simulink model "ECS_FOS"  (Simulink 8.2)
settings: Solver=ode45  StartTime=0.0  StopTime=18000  RelTol=1e-3
InitFcn:
  | load('loss_coeff_mixing_junction.mat')
  | load('SampleOutput.mat')
  | load('HydProp.mat')
  | load('HydraulicLoad.mat')
  | load('initavload.mat')
  | load('SampleFuelBurn.mat')
values from neighbouring files (symbols this model uses):
  FuelBurn = [0 0 0 0 0 0 0 0 0 0 0 0 ... (18249 elements, 1x18249)]    [Benchmark_data1.mat]
  fueltankdata =     [Benchmark_data1.mat]
undefined symbols (not defined in the file or in its folder): AirProp, F1, F2, HUGHES_TREITLER, magnitude, PN_70147, PumpProp
libraries: PowerFlowLib x46, simulink x4
(part 3 of 5)

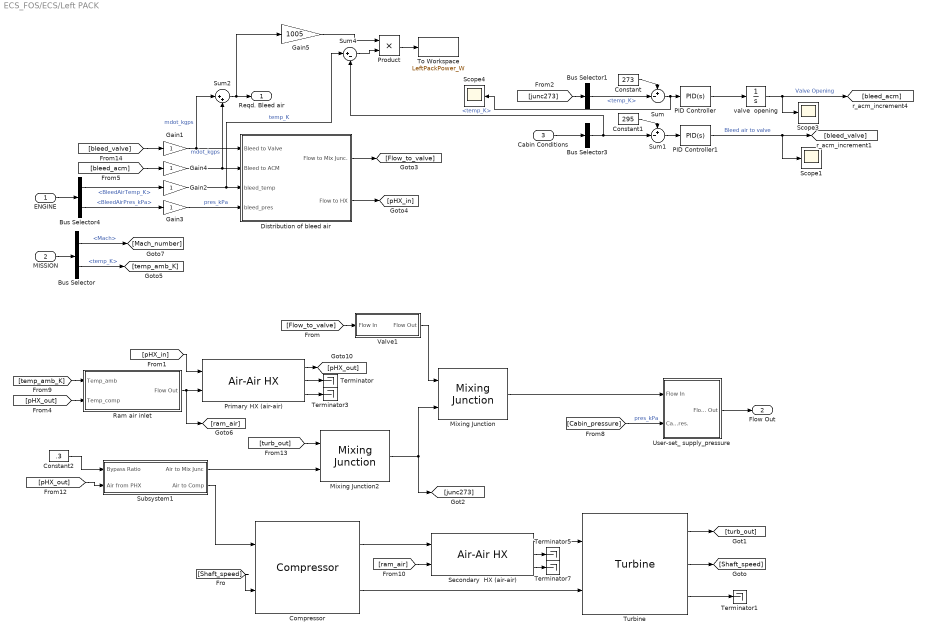
== system ECS_FOS/ECS/Left PACK ==
  ENGINE : Inport
  MISSION : Inport  Port=2
  Cabin Conditions : Inport  Port=3
  Bus Selector : BusSelector  OutputSignals=Flight parameters.Mach,Flight parameters.temp_K
  Bus Selector1 : BusSelector  OutputSignals=temp_K
  Bus Selector3 : BusSelector  OutputSignals=temp_K
  Bus Selector4 : BusSelector  OutputSignals=Bleed.BleedAirTemp_K,Bleed.BleedAirPres_kPa
  Compressor : PowerFlowLib/Energy & Power Systems/Thermal/ECS/Compressor
  Constant : Constant  Value=273
  Constant1 : Constant  Value=295
  Constant2 : Constant  Value=.3
  Distribution of bleed air : Subsystem
      mask Display:
      | port_label('input',1,'{ \bfBleed air to valve [kg/s]}','texmode','on')
      | port_label('input',2,'{ \bfBleed air to ACM [kg/s]}','texmode','on')
      | port_label('input',3,'{ \bfBleed temp. (K)}','texmode','on');
      | port_label('input',4,'{ \bfBleed pressure. (kPa)}','texmode','on')
      | 
      | 
      | 
      | port_label('output',1,'{\bfFlow to Mix Junc. }','texmode','on')
      | port_label('output',2,'{\bfFlow to ACM }','texmode','on')
  Gain{1..4} (4 alike) : Gain
  Gain5 : Gain  Gain=1005
  Mixing Junction : PowerFlowLib/Energy & Power Systems/Thermal/ECS/Mixing Junction  d_in_1=0.1  d_in_2=0.1  d_out=0.2
  Mixing Junction2 : PowerFlowLib/Energy & Power Systems/Thermal/ECS/Mixing Junction  d_in_1=0.1  d_in_2=0.1  d_out=0.2
  PID Controller : simulink/Continuous/PID Controller  Controller=PID  TimeDomain=Continuous-time  SampleTime=1  IntegratorMethod=Forward Euler  FilterMethod=Forward Euler  Form=Parallel  P=.01  I=0  D=0  N=100  InitialConditionSource=internal  InitialConditionForIntegrator=0  InitialConditionForFilter=0  ExternalReset=none  LimitOutput=off  UpperSaturationLimit=inf  LowerSaturationLimit=-inf  LinearizeAsGain=off  AntiWindupMode=none  Kb=1  TrackingMode=off  Kt=1  PParamMin=[]  PParamMax=[]  IParamMin=[]  IParamMax=[]  DParamMin=[]  DParamMax=[]  NParamMin=[]  NParamMax=[]  KbParamMin=[]  KbParamMax=[]  KtParamMin=[]  KtParamMax=[]  POutMin=[]  POutMax=[]  IOutMin=[]  IOutMax=[]  DOutMin=[]  DOutMax=[]  NOutMin=[]  NOutMax=[]  KbOutMin=[]  KbOutMax=[]  KtOutMin=[]  KtOutMax=[]  IntegratorOutMin=[]  IntegratorOutMax=[]  FilterOutMin=[]  FilterOutMax=[]  SumOutMin=[]  SumOutMax=[]  SumI1OutMin=[]  SumI1OutMax=[]  SumI2OutMin=[]  SumI2OutMax=[]  SumI3OutMin=[]  SumI3OutMax=[]  SumDOutMin=[]  SumDOutMax=[]  SaturationOutMin=[]  SaturationOutMax=[]  IntegratorContinuousStateAttributes=''  IntegratorStateMustResolveToSignalObject=off  IntegratorRTWStateStorageClass=Auto  FilterContinuousStateAttributes=''  FilterStateMustResolveToSignalObject=off  FilterRTWStateStorageClass=Auto
  PID Controller1 : simulink/Continuous/PID Controller  Controller=PID  TimeDomain=Continuous-time  SampleTime=1  IntegratorMethod=Forward Euler  FilterMethod=Forward Euler  Form=Parallel  P=.2  I=.01  D=0  N=100  InitialConditionSource=internal  InitialConditionForIntegrator=0  InitialConditionForFilter=0  ExternalReset=none  LimitOutput=on  UpperSaturationLimit=inf  LowerSaturationLimit=.05  LinearizeAsGain=off  AntiWindupMode=none  Kb=1  TrackingMode=off  Kt=1  PParamMin=[]  PParamMax=[]  IParamMin=[]  IParamMax=[]  DParamMin=[]  DParamMax=[]  NParamMin=[]  NParamMax=[]  KbParamMin=[]  KbParamMax=[]  KtParamMin=[]  KtParamMax=[]  POutMin=[]  POutMax=[]  IOutMin=[]  IOutMax=[]  DOutMin=[]  DOutMax=[]  NOutMin=[]  NOutMax=[]  KbOutMin=[]  KbOutMax=[]  KtOutMin=[]  KtOutMax=[]  IntegratorOutMin=[]  IntegratorOutMax=[]  FilterOutMin=[]  FilterOutMax=[]  SumOutMin=[]  SumOutMax=[]  SumI1OutMin=[]  SumI1OutMax=[]  SumI2OutMin=[]  SumI2OutMax=[]  SumI3OutMin=[]  SumI3OutMax=[]  SumDOutMin=[]  SumDOutMax=[]  SaturationOutMin=[]  SaturationOutMax=[]  IntegratorContinuousStateAttributes=''  IntegratorStateMustResolveToSignalObject=off  IntegratorRTWStateStorageClass=Auto  FilterContinuousStateAttributes=''  FilterStateMustResolveToSignalObject=off  FilterRTWStateStorageClass=Auto
  Primary HX (air-air) : PowerFlowLib/Energy & Power Systems/Thermal/ECS/Air-Air HX  L_hx=0.2  W_hx=0.2  H_hx=0.2  t_p=0.0008  K_p=167  cp_hx=883  m_cm=16  l_fin=.005  t_fin=0.0002  s_fin=0.0015  h_fin=0.0095  K_n=167  eta_f=0.8  T_cm_0=50
  Product : Product
  Ram air inlet : Subsystem  mask{ram_air=.5, T_35=273}
      mask prompts: ram_air "Ram air mass flow rate"; T_35 "Temperature control for 35F valve"
      mask Display:
      | port_label('input',1,'{ \bf Ambient Temp.}','texmode','on')
      | port_label('input',2,'{ \bf Comp. Face Temp.}','texmode','on');
      | 
      | port_label('output',1,'{\bf Flow Out}','texmode','on')
  Scope1 : Scope
      settings: YMin=0  YMax=6.5  SaveName=ScopeData33  SampleInput=on  SampleTime=1
  Scope3 : Scope
      settings: YMin=0.735  YMax=0.8  SaveName=ScopeData35  SampleInput=on  SampleTime=1
  Scope4 : Scope
      settings: TimeRange=1500  YMin=2.8421709427e-013  YMax=2.8421709434e-013  SaveName=ScopeData37  SampleInput=on  SampleTime=1
  Secondary  HX (air-air) : PowerFlowLib/Energy & Power Systems/Thermal/ECS/Air-Air HX  L_hx=0.2  W_hx=0.2  H_hx=0.2  t_p=0.0008  K_p=167  cp_hx=883  m_cm=16  l_fin=.005  t_fin=0.0002  s_fin=0.0015  h_fin=0.0095  K_n=167  eta_f=0.8  T_cm_0=25
  Subsystem1 : Subsystem
  Sum : Sum  Inputs=+-|
  Sum1 : Sum  Inputs=+-|
  Sum2 : Sum  Inputs=|++
  Sum4 : Sum  Inputs=|+-
  Terminator{,1,3,5,7} (5 alike) : Terminator
  To Workspace : ToWorkspace  VariableName=LeftPackPower_W  SampleTime=10  SaveFormat=Structure With Time
  Turbine : PowerFlowLib/Energy & Power Systems/Thermal/ECS/Turbine  press_Turbine_exit=80  inertia=5e-5  n_t=0.7
  User-set_ supply_pressure : Subsystem
  Valve1 : Subsystem
  valve  opening : Integrator  InitialCondition=.2  LimitOutput=on  UpperSaturationLimit=.9  LowerSaturationLimit=.2
  Reqd. Bleed air : Outport
  Flow Out : Outport  Port=2
  wires:
  Product/1 -> To Workspace/1
  Sum4/1 -> Product/2
  Gain5/1 -> Product/1
  Constant2/1 -> Subsystem1/1(Bypass Ratio)
  [bleed_acm] -> Gain4/1
  Cabin Conditions/1 -> Bus Selector3/1
  Sum2/1 -> Reqd. Bleed air/1, Gain5/1
  Gain4/1 -> Sum2/2, Distribution of bleed air/2(Bleed to ACM)  "mdot_kgps"
  Constant/1 -> Sum/1
  valve  opening/1 -> [bleed_acm], Scope3/1  "Valve Opening"
  PID Controller/1 -> valve  opening/1
  Sum/1 -> Scope4/1, PID Controller/1
  Bus Selector1/1 -> Sum/2  "<temp_K>"
  [junc273] -> Bus Selector1/1
  Subsystem1/2(Air to Comp) -> Compressor/1
  Subsystem1/1(Air to Mix Junc) -> Mixing Junction2/2
  [turb_out] -> Mixing Junction2/1
  Mixing Junction2/1 -> Mixing Junction/2, [junc273]
  [pHX_out] -> Subsystem1/2(Air from PHX)
  Secondary  HX (air-air)/1 -> Turbine/1
  Secondary  HX (air-air)/3 -> Terminator7/1
  Secondary  HX (air-air)/2 -> Terminator5/1
  Primary HX (air-air)/1 -> [pHX_out]
  Primary HX (air-air)/2 -> Terminator/1
  Primary HX (air-air)/3 -> Terminator3/1
  [bleed_valve] -> Gain1/1
  Gain3/1 -> Distribution of bleed air/4(bleed_pres)  "pres_kPa"
  Gain2/1 -> Distribution of bleed air/3(bleed_temp), Sum4/1  "temp_K"
  Gain1/1 -> Sum2/1, Distribution of bleed air/1(Bleed to Valve)  "mdot_kgps"
  Bus Selector/1 -> [Mach_number]  "<Mach>"
  Bus Selector/2 -> [temp_amb_K]  "<temp_K>"
  Bus Selector4/2 -> Gain3/1  "<BleedAirPres_kPa>"
  Bus Selector4/1 -> Gain2/1  "<BleedAirTemp_K>"
  Distribution of bleed air/1(Flow to Mix Junc.) -> [Flow_to_valve]
  Distribution of bleed air/2(Flow to HX) -> [pHX_in]
  ENGINE/1 -> Bus Selector4/1
  MISSION/1 -> Bus Selector/1
  [pHX_out] -> Ram air inlet/2(Temp_comp)
  [temp_amb_K] -> Ram air inlet/1(Temp_amb)
  [Cabin_pressure] -> User-set_ supply_pressure/2(Cabin Pres.)  "pres_kPa"
  User-set_ supply_pressure/1(Flow Out) -> Flow Out/1
  Turbine/1 -> [turb_out]
  Turbine/3 -> Terminator1/1
  Turbine/2 -> [Shaft_speed]
  Mixing Junction/1 -> User-set_ supply_pressure/1(Flow In)
  [ram_air] -> Secondary  HX (air-air)/2
  Compressor/1 -> Secondary  HX (air-air)/1
  Ram air inlet/1(Flow Out) -> [ram_air], Primary HX (air-air)/2
  Compressor/2 -> Turbine/2
  [Shaft_speed] -> Compressor/2
  [Flow_to_valve] -> Valve1/1(Flow In)
  Valve1/1(Flow Out) -> Mixing Junction/1
  [pHX_in] -> Primary HX (air-air)/1
  Bus Selector3/1 -> Sum1/2, Sum4/2  "<temp_K>"
  Sum1/1 -> PID Controller1/1
  PID Controller1/1 -> Scope1/1, [bleed_valve]  "Bleed air to valve"
  Constant1/1 -> Sum1/1

== system ECS_FOS/ECS/Oil Tanks/Pumps Left Wing ==
  Oil Sys Pres : Inport
  Flow In : Inport  Port=2
  Bus Selector1 : BusSelector  OutputSignals=Oil
  Bus Selector2 : BusSelector  OutputSignals=real_pwr_W,react_pwr_VAr
  Bus Selector5 : BusSelector  OutputSignals=mdot_kgps,pres_kPa
  ElectricalSink1 : PowerFlowLib/Support Functions//Tools/ElectricalSink  Tag=Flow  Description=TwoPhase  load_loc=LeftWing  ACDC_load=AC  units=Watts  unq_id=9405
  Fuel Switch1 : Constant  Value=100
  Fuel Switch2 : Constant  Value=1400
  Fuel Switch3 : Constant  Value=[10 10 10 10 10 10]
  Oil Pump : PowerFlowLib/Energy & Power Systems/Thermal/Oil/Oil Pump  maptype=Pressure (kPa) vs. Vol. Flow Rate (m³/hr)  map=B737_mech_fuel1  map_load=off  SG=0.82  pump_eff=.75  heat_out=off  AC_pwr=on  pf=1  mech_pwr=off
  Oil Tank : Subsystem  AncestorBlock=PowerFlowLib/Energy & Power Systems/Thermal/Fuel/Fuel Tank  mask(Fuel Tank){fileslct=off, filename=fueltank_area.m, filedir=C:\Users\mwillms4\Documents\My Box Files\Graduate\Research\PowerFlow Development\PowerFlow Fall 2013\SupportFunctions\fueltank_area.m, tank_loc=Left Wing Tank, areaprompt2=off, max_vol=3.2, m_init=2500, fld_Tint=0, ull_Tint=30, Pover=100, HTC_fg=14.2, wallHXF=off, wetHTC=14.2, dryHTC=14.2, Qinternal=0}
      mask prompts: fileslct "Browse for area .m file?"; filename "Fuel Tank Area .m File"; filedir "Area .m File Directory"; tank_loc "Select Tank"; areaprompt2 "Edit Fuel Tank Area Manually?"; max_vol "Maximum Tank Volume [m³]"; m_init "Initial Fluid Mass [kg]"; fld_Tint "Initial Fluid Temperature [°C]"; ull_Tint "Initial Ullage Temperature [°C]"; Pover "Tank Pressurization [kPa]"; HTC_fg "Fuel to Ullage HTC [W/m² K]"; wallHXF "Enable Wall Heat Transfer"; wetHTC "Wall to Fluid HTC [W/m² K]"; dryHTC "Wall to Ullage HTC [W/m² K]"; Qinternal "Internal Heat Load [W]"
      mask help:
      | Input 1: Input Flow Bus
      | Input 2: Flow Rate Out [kg/s]
      | Input 3: Ambient Pressure [kPa]
      | Input 4: Heat Load [W]
      | Input 5: Initial Wall Temps. Vector [K]
      |
      | Output 1: Output Flow Bus
      | Output 2: Tank mass [kg]
      | Output 3: Ullage Temp. [K]
      mask init: same as ECS_FOS/ECS/Fuel Tanks/Pumps/Center Fuel Tank
      mask Callback fileslct:
      | h      = get_param(gcb,'handle');   % Get block handle
      | blk    = gcb;
      | hblock = get(h);     % Parse out handles structure
      | 
      | if strcmp(hblock.fileslct,'on') == 1;
      |     set_param(gcb,'areaprompt2','off');     % turn off manual switch
      |     RR_SetPerfSlct(2,0);                    % call uiopen script
      | end
      | 
      | clear h blk hblock
      mask TypeOptions tank_loc: Left Wing Tank | Center Tank | Right Wing Tank
      mask Callback areaprompt2:
      | h      = get_param(gcb,'handle');   % Get block handle
      | blk    = gcb;
      | hblock = get(h);     % Parse out handles structure
      | 
      | if strcmp(hblock.areaprompt2,'on') == 1;
      |     set_param(gcb,'fileslct','off');
      |     open_system([blk, '/Wall Heat Transfer/volume_%']);
      | end
      mask Callback wallHXF:
      | h      = get_param(gcb,'handle');   % Get block handle
      | blk    = gcb;
      | hblock = get(h);     % Parse out handles structure
      | 
      | if strcmp(hblock.wallHXF,'on') == 1;
      |     set_param([blk,'/enable_wall_HXF'],'Value','1');
      | else
      |     set_param([blk,'/enable_wall_HXF'],'Value','0');
      | end
      | 
      | clear h blk hblock
      mask Display:
      | image(imread('fueltank.jpg'))
      | 
      | port_label('input',1,'{\bf Flow In}','TexMode','on')
      | port_label('input',2,'{\bf Flow Rate Out}','TexMode','on')
      | port_label('input',3,'{\bf P_a_m_b [kPa]}','TexMode','on')
      | port_label('input',4,'{\bf Heat Load [kW]}','TexMode','on')
      | port_label('input',5,'{\bf Wall Temp. [K]}','TexMode','on')
      | 
      | port_label('output',1,'{\bf Flow Out }','TexMode','on')
      | port_label('output',2,'{\bf Fluid Mass [kg]}','TexMode','on')
      | port_label('output',3,'{\bf Ullage Temp. [K]}','TexMode','on')
  Terminator : Terminator
  Terminator1 : Terminator
  Oil To HX : Outport
  wires:
  Oil Pump/2 -> Bus Selector2/1
  Bus Selector2/2 -> ElectricalSink1/2  "<react_pwr_VAr>"
  Bus Selector2/1 -> ElectricalSink1/1  "<real_pwr_W>"
  Oil Tank/1(Flow_Out) -> Oil Pump/1
  Oil Tank/2(fluid_mass) -> Terminator/1
  Oil Tank/3(ullage_T) -> Terminator1/1
  Fuel Switch3/1 -> Oil Tank/5(Wall_temps)
  Oil Pump/3 -> Oil Tank/4(Heat load)
  Oil Pump/1 -> Bus Selector5/1, Oil To HX/1
  Fuel Switch1/1 -> Oil Tank/3(Pamb)
  Oil Sys Pres/1 -> Oil Pump/3
  Flow In/1 -> Bus Selector1/1
  Fuel Switch2/1 -> Oil Pump/2
  Bus Selector5/1 -> Oil Tank/2(Flow Out)  "<mdot_kgps>"
  Bus Selector1/1 -> Oil Tank/1(Flow)  "<Oil>"

== system ECS_FOS/ECS/Oil Tanks/Pumps Right Wing ==
  Oil Sys Pres : Inport
  Flow In : Inport  Port=2
  Bus Selector1 : BusSelector  OutputSignals=Oil
  Bus Selector2 : BusSelector  OutputSignals=real_pwr_W,react_pwr_VAr
  Bus Selector5 : BusSelector  OutputSignals=mdot_kgps,pres_kPa
  ElectricalSink1 : PowerFlowLib/Support Functions//Tools/ElectricalSink  Tag=Flow  Description=TwoPhase  load_loc=RightWing  ACDC_load=AC  units=Watts  unq_id=2169
  Fuel Switch2 : Constant  Value=1400
  Fuel Tank : Subsystem  AncestorBlock=PowerFlowLib/Energy & Power Systems/Thermal/Fuel/Fuel Tank  mask(Fuel Tank){fileslct=off, filename=fueltank_area.m, filedir=C:\Users\mwillms4\Documents\My Box Files\Graduate\Research\PowerFlow Development\PowerFlow Fall 2013\SupportFunctions\fueltank_area.m, tank_loc=Left Wing Tank, areaprompt2=off, max_vol=3.2, m_init=2500, fld_Tint=0, ull_Tint=30, Pover=100, HTC_fg=14.2, wallHXF=off, wetHTC=14.2, dryHTC=14.2, Qinternal=0}
      mask prompts: fileslct "Browse for area .m file?"; filename "Fuel Tank Area .m File"; filedir "Area .m File Directory"; tank_loc "Select Tank"; areaprompt2 "Edit Fuel Tank Area Manually?"; max_vol "Maximum Tank Volume [m³]"; m_init "Initial Fluid Mass [kg]"; fld_Tint "Initial Fluid Temperature [°C]"; ull_Tint "Initial Ullage Temperature [°C]"; Pover "Tank Pressurization [kPa]"; HTC_fg "Fuel to Ullage HTC [W/m² K]"; wallHXF "Enable Wall Heat Transfer"; wetHTC "Wall to Fluid HTC [W/m² K]"; dryHTC "Wall to Ullage HTC [W/m² K]"; Qinternal "Internal Heat Load [W]"
      mask help:
      | Input 1: Input Flow Bus
      | Input 2: Flow Rate Out [kg/s]
      | Input 3: Ambient Pressure [kPa]
      | Input 4: Heat Load [W]
      | Input 5: Initial Wall Temps. Vector [K]
      |
      | Output 1: Output Flow Bus
      | Output 2: Tank mass [kg]
      | Output 3: Ullage Temp. [K]
      mask init: same as ECS_FOS/ECS/Fuel Tanks/Pumps/Center Fuel Tank
      mask Callback fileslct:
      | h      = get_param(gcb,'handle');   % Get block handle
      | blk    = gcb;
      | hblock = get(h);     % Parse out handles structure
      | 
      | if strcmp(hblock.fileslct,'on') == 1;
      |     set_param(gcb,'areaprompt2','off');     % turn off manual switch
      |     RR_SetPerfSlct(2,0);                    % call uiopen script
      | end
      | 
      | clear h blk hblock
      mask TypeOptions tank_loc: Left Wing Tank | Center Tank | Right Wing Tank
      mask Callback areaprompt2:
      | h      = get_param(gcb,'handle');   % Get block handle
      | blk    = gcb;
      | hblock = get(h);     % Parse out handles structure
      | 
      | if strcmp(hblock.areaprompt2,'on') == 1;
      |     set_param(gcb,'fileslct','off');
      |     open_system([blk, '/Wall Heat Transfer/volume_%']);
      | end
      mask Callback wallHXF:
      | h      = get_param(gcb,'handle');   % Get block handle
      | blk    = gcb;
      | hblock = get(h);     % Parse out handles structure
      | 
      | if strcmp(hblock.wallHXF,'on') == 1;
      |     set_param([blk,'/enable_wall_HXF'],'Value','1');
      | else
      |     set_param([blk,'/enable_wall_HXF'],'Value','0');
      | end
      | 
      | clear h blk hblock
      mask Display:
      | image(imread('fueltank.jpg'))
      | 
      | port_label('input',1,'{\bf Flow In}','TexMode','on')
      | port_label('input',2,'{\bf Flow Rate Out}','TexMode','on')
      | port_label('input',3,'{\bf P_a_m_b [kPa]}','TexMode','on')
      | port_label('input',4,'{\bf Heat Load [kW]}','TexMode','on')
      | port_label('input',5,'{\bf Wall Temp. [K]}','TexMode','on')
      | 
      | port_label('output',1,'{\bf Flow Out }','TexMode','on')
      | port_label('output',2,'{\bf Fluid Mass [kg]}','TexMode','on')
      | port_label('output',3,'{\bf Ullage Temp. [K]}','TexMode','on')
  Ground : Ground
  Ground1 : Ground
  Oil Pump : PowerFlowLib/Energy & Power Systems/Thermal/Oil/Oil Pump  maptype=Pressure (kPa) vs. Vol. Flow Rate (m³/hr)  map=B737_mech_fuel1  map_load=off  SG=0.82  pump_eff=.75  heat_out=off  AC_pwr=on  pf=1  mech_pwr=off
  Terminator : Terminator
  Terminator1 : Terminator
  Oil To HX : Outport
  wires:
  Bus Selector1/1 -> Fuel Tank/1(Flow)  "<Oil>"
  Oil Pump/2 -> Bus Selector2/1
  Bus Selector2/2 -> ElectricalSink1/2  "<react_pwr_VAr>"
  Bus Selector2/1 -> ElectricalSink1/1  "<real_pwr_W>"
  Bus Selector5/1 -> Fuel Tank/2(Flow Out)  "<mdot_kgps>"
  Fuel Switch2/1 -> Oil Pump/2
  Flow In/1 -> Bus Selector1/1
  Oil Sys Pres/1 -> Oil Pump/3
  Ground1/1 -> Fuel Tank/3(Pamb)
  Oil Pump/1 -> Oil To HX/1, Bus Selector5/1
  Oil Pump/3 -> Fuel Tank/4(Heat load)
  Ground/1 -> Fuel Tank/5(Wall_temps)
  Fuel Tank/3(ullage_T) -> Terminator1/1
  Fuel Tank/2(fluid_mass) -> Terminator/1
  Fuel Tank/1(Flow_Out) -> Oil Pump/1

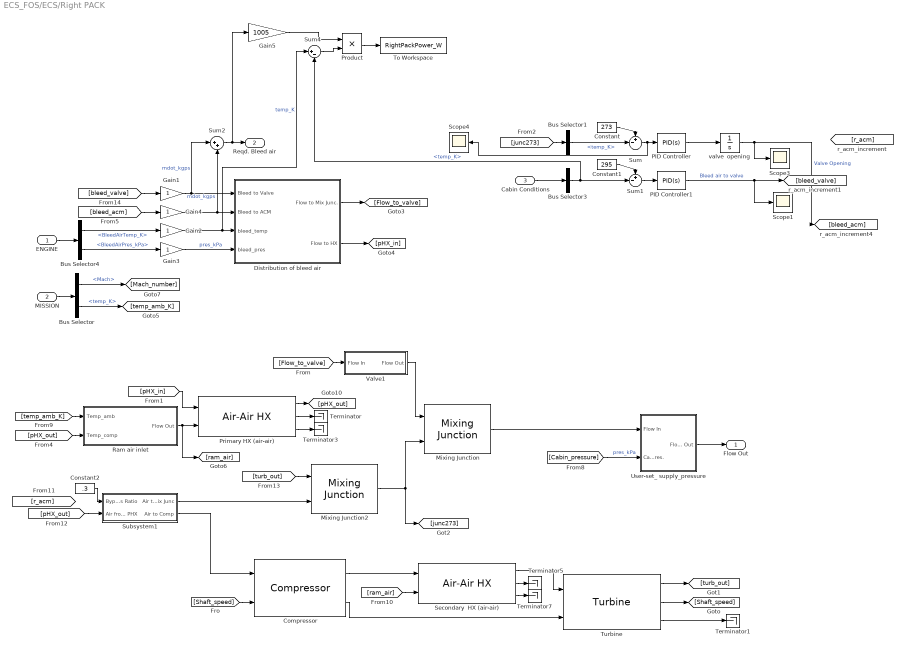
== system ECS_FOS/ECS/Right PACK ==
  ENGINE : Inport
  MISSION : Inport  Port=2
  Cabin Conditions : Inport  Port=3
  Bus Selector : BusSelector  OutputSignals=Flight parameters.Mach,Flight parameters.temp_K
  Bus Selector1 : BusSelector  OutputSignals=temp_K
  Bus Selector3 : BusSelector  OutputSignals=temp_K
  Bus Selector4 : BusSelector  OutputSignals=Bleed.BleedAirTemp_K,Bleed.BleedAirPres_kPa
  Compressor : PowerFlowLib/Energy & Power Systems/Thermal/ECS/Compressor
  Constant : Constant  Value=273
  Constant1 : Constant  Value=295
  Constant2 : Constant  Value=.3
  Distribution of bleed air : Subsystem
      mask Display:
      | port_label('input',1,'{ \bfBleed air to valve [kg/s]}','texmode','on')
      | port_label('input',2,'{ \bfBleed air to ACM [kg/s]}','texmode','on')
      | port_label('input',3,'{ \bfBleed temp. (K)}','texmode','on');
      | port_label('input',4,'{ \bfBleed pressure. (kPa)}','texmode','on')
      | 
      | 
      | 
      | port_label('output',1,'{\bfFlow to Mix Junc. }','texmode','on')
      | port_label('output',2,'{\bfFlow to ACM }','texmode','on')
  Gain{1..4} (4 alike) : Gain
  Gain5 : Gain  Gain=1005
  Mixing Junction : PowerFlowLib/Energy & Power Systems/Thermal/ECS/Mixing Junction  d_in_1=0.1  d_in_2=0.1  d_out=0.2
  Mixing Junction2 : PowerFlowLib/Energy & Power Systems/Thermal/ECS/Mixing Junction  d_in_1=0.1  d_in_2=0.1  d_out=0.2
  PID Controller : simulink/Continuous/PID Controller  Controller=PID  TimeDomain=Continuous-time  SampleTime=1  IntegratorMethod=Forward Euler  FilterMethod=Forward Euler  Form=Parallel  P=.01  I=0  D=0  N=100  InitialConditionSource=internal  InitialConditionForIntegrator=0  InitialConditionForFilter=0  ExternalReset=none  LimitOutput=off  UpperSaturationLimit=inf  LowerSaturationLimit=-inf  LinearizeAsGain=off  AntiWindupMode=none  Kb=1  TrackingMode=off  Kt=1  PParamMin=[]  PParamMax=[]  IParamMin=[]  IParamMax=[]  DParamMin=[]  DParamMax=[]  NParamMin=[]  NParamMax=[]  KbParamMin=[]  KbParamMax=[]  KtParamMin=[]  KtParamMax=[]  POutMin=[]  POutMax=[]  IOutMin=[]  IOutMax=[]  DOutMin=[]  DOutMax=[]  NOutMin=[]  NOutMax=[]  KbOutMin=[]  KbOutMax=[]  KtOutMin=[]  KtOutMax=[]  IntegratorOutMin=[]  IntegratorOutMax=[]  FilterOutMin=[]  FilterOutMax=[]  SumOutMin=[]  SumOutMax=[]  SumI1OutMin=[]  SumI1OutMax=[]  SumI2OutMin=[]  SumI2OutMax=[]  SumI3OutMin=[]  SumI3OutMax=[]  SumDOutMin=[]  SumDOutMax=[]  SaturationOutMin=[]  SaturationOutMax=[]  IntegratorContinuousStateAttributes=''  IntegratorStateMustResolveToSignalObject=off  IntegratorRTWStateStorageClass=Auto  FilterContinuousStateAttributes=''  FilterStateMustResolveToSignalObject=off  FilterRTWStateStorageClass=Auto
  PID Controller1 : simulink/Continuous/PID Controller  Controller=PID  TimeDomain=Continuous-time  SampleTime=1  IntegratorMethod=Forward Euler  FilterMethod=Forward Euler  Form=Parallel  P=.2  I=.01  D=0  N=0  InitialConditionSource=internal  InitialConditionForIntegrator=0  InitialConditionForFilter=0  ExternalReset=none  LimitOutput=on  UpperSaturationLimit=10  LowerSaturationLimit=.05  LinearizeAsGain=off  AntiWindupMode=none  Kb=1  TrackingMode=off  Kt=1  PParamMin=[]  PParamMax=[]  IParamMin=[]  IParamMax=[]  DParamMin=[]  DParamMax=[]  NParamMin=[]  NParamMax=[]  KbParamMin=[]  KbParamMax=[]  KtParamMin=[]  KtParamMax=[]  POutMin=[]  POutMax=[]  IOutMin=[]  IOutMax=[]  DOutMin=[]  DOutMax=[]  NOutMin=[]  NOutMax=[]  KbOutMin=[]  KbOutMax=[]  KtOutMin=[]  KtOutMax=[]  IntegratorOutMin=[]  IntegratorOutMax=[]  FilterOutMin=[]  FilterOutMax=[]  SumOutMin=[]  SumOutMax=[]  SumI1OutMin=[]  SumI1OutMax=[]  SumI2OutMin=[]  SumI2OutMax=[]  SumI3OutMin=[]  SumI3OutMax=[]  SumDOutMin=[]  SumDOutMax=[]  SaturationOutMin=[]  SaturationOutMax=[]  IntegratorContinuousStateAttributes=''  IntegratorStateMustResolveToSignalObject=off  IntegratorRTWStateStorageClass=Auto  FilterContinuousStateAttributes=''  FilterStateMustResolveToSignalObject=off  FilterRTWStateStorageClass=Auto
  Primary HX (air-air) : PowerFlowLib/Energy & Power Systems/Thermal/ECS/Air-Air HX  L_hx=0.2  W_hx=0.2  H_hx=0.2  t_p=0.0008  K_p=167  cp_hx=883  m_cm=16  l_fin=.005  t_fin=0.0002  s_fin=0.0015  h_fin=0.0095  K_n=167  eta_f=0.8  T_cm_0=50
  Product : Product
  Ram air inlet : Subsystem  mask{ram_air=.5, T_35=273}
      mask prompts: ram_air "Ram air mass flow rate"; T_35 "Temperature control for 35F valve"
      mask Display:
      | port_label('input',1,'{ \bf Ambient Temp.}','texmode','on')
      | port_label('input',2,'{ \bf Comp. Face Temp.}','texmode','on');
      | 
      | port_label('output',1,'{\bf Flow Out}','texmode','on')
  Scope1 : Scope
      settings: YMin=0  YMax=6.5  SaveName=ScopeData33  SampleInput=on  SampleTime=1
  Scope3 : Scope
      settings: YMin=0.427  YMax=0.437  SaveName=ScopeData35  SampleInput=on  SampleTime=1
  Scope4 : Scope
      settings: YMin=0.048825  YMax=0.04905  SaveName=ScopeData37  SampleInput=on  SampleTime=1
  Secondary  HX (air-air) : PowerFlowLib/Energy & Power Systems/Thermal/ECS/Air-Air HX  L_hx=0.2  W_hx=0.2  H_hx=0.2  t_p=0.0008  K_p=167  cp_hx=883  m_cm=16  l_fin=.005  t_fin=0.0002  s_fin=0.0015  h_fin=0.0095  K_n=167  eta_f=0.8  T_cm_0=25
  Subsystem1 : Subsystem
  Sum : Sum  Inputs=+-|
  Sum1 : Sum  Inputs=+-|
  Sum2 : Sum  Inputs=|++
  Sum4 : Sum  Inputs=|+-
  Terminator{,1,3,5,7} (5 alike) : Terminator
  To Workspace : ToWorkspace  VariableName=RightPackPower_W  SampleTime=10  SaveFormat=Structure With Time
  Turbine : PowerFlowLib/Energy & Power Systems/Thermal/ECS/Turbine  press_Turbine_exit=80  inertia=5e-5  n_t=0.7
  User-set_ supply_pressure : Subsystem
  Valve1 : Subsystem
  valve  opening : Integrator  InitialCondition=.5  LimitOutput=on  UpperSaturationLimit=0.8  LowerSaturationLimit=0.2
  Flow Out : Outport
  Reqd. Bleed air : Outport  Port=2
  wires:
  Product/1 -> To Workspace/1
  Sum4/1 -> Product/2
  Gain5/1 -> Product/1
  Sum2/1 -> Reqd. Bleed air/1, Gain5/1
  Gain2/1 -> Distribution of bleed air/3(bleed_temp), Sum4/1  "temp_K"
  Bus Selector3/1 -> Sum1/2, Sum4/2  "<temp_K>"
  Constant2/1 -> Subsystem1/1(Bypass Ratio)
  [bleed_acm] -> Gain4/1
  Constant1/1 -> Sum1/1
  PID Controller1/1 -> [bleed_valve], Scope1/1  "Bleed air to valve"
  Sum1/1 -> PID Controller1/1
  [pHX_in] -> Primary HX (air-air)/1
  Valve1/1(Flow Out) -> Mixing Junction/1
  [Flow_to_valve] -> Valve1/1(Flow In)
  [Shaft_speed] -> Compressor/2
  Compressor/2 -> Turbine/2
  Ram air inlet/1(Flow Out) -> Primary HX (air-air)/2, [ram_air]
  Compressor/1 -> Secondary  HX (air-air)/1
  [ram_air] -> Secondary  HX (air-air)/2
  Mixing Junction/1 -> User-set_ supply_pressure/1(Flow In)
  Turbine/2 -> [Shaft_speed]
  Turbine/3 -> Terminator1/1
  Turbine/1 -> [turb_out]
  User-set_ supply_pressure/1(Flow Out) -> Flow Out/1
  [Cabin_pressure] -> User-set_ supply_pressure/2(Cabin Pres.)  "pres_kPa"
  [temp_amb_K] -> Ram air inlet/1(Temp_amb)
  [pHX_out] -> Ram air inlet/2(Temp_comp)
  MISSION/1 -> Bus Selector/1
  ENGINE/1 -> Bus Selector4/1
  Distribution of bleed air/2(Flow to HX) -> [pHX_in]
  Distribution of bleed air/1(Flow to Mix Junc.) -> [Flow_to_valve]
  Bus Selector4/1 -> Gain2/1  "<BleedAirTemp_K>"
  Bus Selector4/2 -> Gain3/1  "<BleedAirPres_kPa>"
  Bus Selector/2 -> [temp_amb_K]  "<temp_K>"
  Bus Selector/1 -> [Mach_number]  "<Mach>"
  Gain1/1 -> Distribution of bleed air/1(Bleed to Valve), Sum2/1  "mdot_kgps"
  Gain3/1 -> Distribution of bleed air/4(bleed_pres)  "pres_kPa"
  [bleed_valve] -> Gain1/1
  Primary HX (air-air)/3 -> Terminator3/1
  Primary HX (air-air)/2 -> Terminator/1
  Primary HX (air-air)/1 -> [pHX_out]
  Secondary  HX (air-air)/2 -> Terminator5/1
  Secondary  HX (air-air)/3 -> Terminator7/1
  Secondary  HX (air-air)/1 -> Turbine/1
  [pHX_out] -> Subsystem1/2(Air from PHX)
  Mixing Junction2/1 -> [junc273], Mixing Junction/2
  [turb_out] -> Mixing Junction2/1
  Subsystem1/1(Air to Mix Junc) -> Mixing Junction2/2
  Subsystem1/2(Air to Comp) -> Compressor/1
  [junc273] -> Bus Selector1/1
  Bus Selector1/1 -> Sum/2  "<temp_K>"
  Sum/1 -> PID Controller/1, Scope4/1
  PID Controller/1 -> valve  opening/1
  valve  opening/1 -> [bleed_acm], Scope3/1  "Valve Opening"
  Constant/1 -> Sum/1
  Gain4/1 -> Distribution of bleed air/2(Bleed to ACM), Sum2/2  "mdot_kgps"
  Cabin Conditions/1 -> Bus Selector3/1

== system ECS_FOS/ECS/Thermal_sources_from Electrical_power_model1 ==
  Gain : Gain
  Terminator : Terminator
  Terminator1 : Terminator
  Terminator2 : Terminator
  ThermalSource : Subsystem  Tag=Flow  Description=TwoPhase  mask(Thermal Source){load_loc=Cockpit}
      mask prompts: load_loc "Location"
      mask help: Output of all thermal loads from the selected location. Loads are in Watts.
      mask init:
      | init_thermal_sourcesink(1)
      settings: CopyFcn=|
      | vals = get_param(gcb,'MaskValues');
      | set_param(gcb,'MaskValues',[vals(1);num2str(0)]);
      mask TypeOptions load_loc: Cockpit | Cabin | CargoBay | LeftWing | RightWing | Empennage
      mask Display:
      | text(.5,.7,'Thermal Source','horizontalAlignment','center','texmode','on')
      | text(.5,.4,get_param(gcb,'load_loc'),'horizontalAlignment','center','texmode','on')
  ThermalSource3 : Subsystem  Tag=Flow  Description=TwoPhase  mask(Thermal Source){load_loc=RightWing}
      mask prompts: load_loc "Location"
      mask help: Output of all thermal loads from the selected location. Loads are in Watts.
      mask init:
      | init_thermal_sourcesink(1)
      settings: CopyFcn=|
      | vals = get_param(gcb,'MaskValues');
      | set_param(gcb,'MaskValues',[vals(1);num2str(0)]);
      mask TypeOptions load_loc: Cockpit | Cabin | CargoBay | LeftWing | RightWing | Empennage
      mask Display:
      | text(.5,.7,'Thermal Source','horizontalAlignment','center','texmode','on')
      | text(.5,.4,get_param(gcb,'load_loc'),'horizontalAlignment','center','texmode','on')
  ThermalSource4 : Subsystem  Tag=Flow  Description=TwoPhase  mask(Thermal Source){load_loc=Empennage}
      mask prompts: load_loc "Location"
      mask help: Output of all thermal loads from the selected location. Loads are in Watts.
      mask init:
      | init_thermal_sourcesink(1)
      settings: CopyFcn=|
      | vals = get_param(gcb,'MaskValues');
      | set_param(gcb,'MaskValues',[vals(1);num2str(0)]);
      mask TypeOptions load_loc: Cockpit | Cabin | CargoBay | LeftWing | RightWing | Empennage
      mask Display:
      | text(.5,.7,'Thermal Source','horizontalAlignment','center','texmode','on')
      | text(.5,.4,get_param(gcb,'load_loc'),'horizontalAlignment','center','texmode','on')
  ThermalSource5 : Subsystem  Tag=Flow  Description=TwoPhase  mask(Thermal Source){load_loc=LeftWing}
      mask prompts: load_loc "Location"
      mask help: Output of all thermal loads from the selected location. Loads are in Watts.
      mask init:
      | init_thermal_sourcesink(1)
      settings: CopyFcn=|
      | vals = get_param(gcb,'MaskValues');
      | set_param(gcb,'MaskValues',[vals(1);num2str(0)]);
      mask TypeOptions load_loc: Cockpit | Cabin | CargoBay | LeftWing | RightWing | Empennage
      mask Display:
      | text(.5,.7,'Thermal Source','horizontalAlignment','center','texmode','on')
      | text(.5,.4,get_param(gcb,'load_loc'),'horizontalAlignment','center','texmode','on')
  Thermal Loads : Outport
  wires:
  ThermalSource5/1(Load) -> Terminator/1
  ThermalSource4/1(Load) -> Terminator2/1
  ThermalSource3/1(Load) -> Terminator1/1
  Gain/1 -> Thermal Loads/1
  ThermalSource/1(Load) -> Gain/1

== system ECS_FOS/Engine #1 - updated 12/1/Heat Loads ==
  Flow In : Inport
  Bus Creator : BusCreator
  Bus Selector : BusSelector  OutputSignals=temp_K,mdot_kgps,pres_kPa,h_kJ/kg
  Gain : Gain  Gain=.1
  Random Number : RandomNumber  Mean=20  Variance=10  SampleTime=0.1
  Sum : Sum  Inputs=++|
  Flow Out : Outport
  wires:
  Flow In/1 -> Bus Selector/1
  Bus Selector/1 -> Sum/2  "<temp_K>"
  Random Number/1 -> Sum/1
  Bus Creator/1 -> Flow Out/1
  Sum/1 -> Bus Creator/1  "temp_K"
  Bus Selector/2 -> Bus Creator/2  "<mdot_kgps>"
  Bus Selector/3 -> Gain/1  "<pres_kPa>"
  Bus Selector/4 -> Bus Creator/4  "<h_kJ/kg>"
  Gain/1 -> Bus Creator/3  "pres_kPa"

== system ECS_FOS/Engine #1 - updated 12/10/Heat Loads ==
  Flow In : Inport
  Bus Creator : BusCreator
  Bus Selector : BusSelector  OutputSignals=temp_K,mdot_kgps,pres_kPa,h_kJ/kg
  Gain : Gain  Gain=.1
  Random Number : RandomNumber  Mean=20  Variance=10  SampleTime=0.1
  Sum : Sum  Inputs=++|
  Flow Out : Outport
  wires:
  Gain/1 -> Bus Creator/3  "pres_kPa"
  Bus Selector/4 -> Bus Creator/4  "<h_kJ/kg>"
  Bus Selector/3 -> Gain/1  "<pres_kPa>"
  Bus Selector/2 -> Bus Creator/2  "<mdot_kgps>"
  Sum/1 -> Bus Creator/1  "temp_K"
  Bus Creator/1 -> Flow Out/1
  Random Number/1 -> Sum/1
  Bus Selector/1 -> Sum/2  "<temp_K>"
  Flow In/1 -> Bus Selector/1

== system ECS_FOS/ECS/Cabin Zone/Air Properties ==
  note: I used the nominal values instead of feading back
      | the cabin temperature and pressure.
  Supply Air : Inport
  Bus Creator{,1..3} (4 alike) : BusCreator  Inputs=3
  Bus Selector : BusSelector  OutputSignals=pres_kPa,temp_K
  Cp(P,T){,1..3} (4 alike) : Lookup_n-D  BreakpointsForDimension1=AirProp.P  BreakpointsForDimension2=AirProp.T  BreakpointsForDimension3=[1]  Table=AirProp.Cp_pt  RndMeth=Simplest  InputSameDT=on
  Nominal cabin press_kPa : Constant  Value=80
  Nominal cabin temp_K : Constant  Value=298
  R_a{1..4} (4 alike) : Constant  Value=287
  Rho(P,T){,1..3} (4 alike) : Lookup_n-D  BreakpointsForDimension1=AirProp.P  BreakpointsForDimension2=AirProp.T  BreakpointsForDimension3=[1]  Table=AirProp.Rho_pt  RndMeth=Simplest  InputSameDT=on
  Supply_AirProp : Outport
  Recirc_AirProp : Outport  Port=2
  Exhaust_AirProp : Outport  Port=3
  Cabin_AirProp : Outport  Port=4
  wires:
  Supply Air/1 -> Bus Selector/1
  Bus Selector/1 -> Rho(P,T)/1, Cp(P,T)/1  "<pres_kPa>"
  Bus Creator/1 -> Supply_AirProp/1
  Bus Creator1/1 -> Recirc_AirProp/1
  Bus Creator2/1 -> Exhaust_AirProp/1
  Bus Creator3/1 -> Cabin_AirProp/1
  Bus Selector/2 -> Cp(P,T)/2, Rho(P,T)/2  "<temp_K>"
  Nominal cabin press_kPa/1 -> Rho(P,T)1/1, Cp(P,T)1/1, Rho(P,T)2/1, Cp(P,T)2/1, Rho(P,T)3/1, Cp(P,T)3/1
  Nominal cabin temp_K/1 -> Rho(P,T)1/2, Cp(P,T)1/2, Rho(P,T)2/2, Cp(P,T)2/2, Rho(P,T)3/2, Cp(P,T)3/2
  R_a4/1 -> Bus Creator/1  "R_a"
  Rho(P,T)/1 -> Bus Creator/2  "Rho_sa"
  Cp(P,T)/1 -> Bus Creator/3  "Cp_sa"
  Rho(P,T)1/1 -> Bus Creator1/2  "Rho_ra"
  Cp(P,T)1/1 -> Bus Creator1/3  "Cp_ra"
  Rho(P,T)2/1 -> Bus Creator2/2  "Rho_ea"
  Cp(P,T)2/1 -> Bus Creator2/3  "Cp_ea"
  Rho(P,T)3/1 -> Bus Creator3/2  "Rho_cab"
  Cp(P,T)3/1 -> Bus Creator3/3  "Cp_cab"
  R_a2/1 -> Bus Creator1/1  "R_a"
  R_a1/1 -> Bus Creator2/1  "R_a"
  R_a3/1 -> Bus Creator3/1  "R_a"

== system ECS_FOS/ECS/Cabin Zone/Cabin Pressurization ==
  Sup. Air mdot : Inport
  Cabin Temp. [C] : Inport  Port=2
  Cabin Prop. : Inport  Port=3
  Cabin Param. : Inport  Port=4
  Bias : Bias  Bias=273.15
  Bus Creator : BusCreator
  Bus Selector : BusSelector  OutputSignals=RAR,V_cab_m^3
  Bus Selector1 : BusSelector  OutputSignals=R_a
  Integrator : Integrator  InitialCondition=122/2
  P_cab_Pa_Ideal_gas_EOS : Product  Inputs=***/
  Pa to kPa : Gain  Gain=1/1000
  Scope : Scope
      settings: SaveName=ScopeData3
  m_dot_ea(assuming no accumulation) : Sum  Inputs=+-
  m_dot_ra : Product  Inputs=**
  net_mass_in : Sum  Inputs=+--
  Cabin mdot & mass : Outport
  Cabin Pres. : Outport  Port=2
  wires:
  Pa to kPa/1 -> Cabin Pres./1  "pres_kPa"
  Bias/1 -> P_cab_Pa_Ideal_gas_EOS/3
  Sup. Air mdot/1 -> m_dot_ra/1, net_mass_in/1, m_dot_ea(assuming no accumulation)/1, Bus Creator/1  "m_dot_sa"
  Cabin Param./1 -> Bus Selector/1
  Bus Selector/1 -> m_dot_ra/2  "<RAR>"
  m_dot_ra/1 -> m_dot_ea(assuming no accumulation)/2, net_mass_in/2, Bus Creator/2  "m_dot_ra"
  m_dot_ea(assuming no accumulation)/1 -> net_mass_in/3, Bus Creator/3  "m_dot_ea"
  net_mass_in/1 -> Integrator/1  "dm_cab/dt"
  Integrator/1 -> Scope/1, Bus Creator/4, P_cab_Pa_Ideal_gas_EOS/1  "m_cab"
  Bus Creator/1 -> Cabin mdot & mass/1
  Cabin Prop./1 -> Bus Selector1/1
  Bus Selector1/1 -> P_cab_Pa_Ideal_gas_EOS/2  "<R_a>"
  Cabin Temp. [C]/1 -> Bias/1  "t_cab_C"
  Bus Selector/2 -> P_cab_Pa_Ideal_gas_EOS/4  "<V_cab_m^3>"
  P_cab_Pa_Ideal_gas_EOS/1 -> Pa to kPa/1

== system ECS_FOS/ECS/Cabin Zone/Cabin Temperature ==
  Sup. Air Temp [C] : Inport
  Cabin mdot & mass : Inport  Port=2
  Cabin Param. : Inport  Port=3
  Air Props. : Inport  Port=4
  Amb Temp [K] : Inport  Port=5
  Mach # : Inport  Port=6
  Add : Sum  Inputs=+++
  Add1 : Sum  Inputs=+-+
  Bus Selector : BusSelector  OutputSignals=m_dot_sa,m_cab,m_dot_ra,m_dot_ea
  Bus Selector1 : BusSelector  OutputSignals=signal2.Cp_sa,signal1.Cp_cab,signal3.Cp_ra,signal4.Cp_ea
  Bus Selector2 : BusSelector  OutputSignals=n_pass,q_pass_W
  Bus Selector3 : BusSelector  OutputSignals=area_m2,U_Wpm2K
  Fuselage_parameters1 : Subsystem
  Integrator : Integrator  InitialCondition=20
  K_to_C : Bias  Bias=-273.15
  Kinetic Heating : Subsystem
  Scope : Scope
  Scope1 : Scope
      settings: SaveName=ScopeData3
  Scope2 : Scope  NumInputPorts=5
      settings: YMin=72~0.1824~1009~57.95~955.7  YMax=85~0.2016~1010~64.05~1056.3  SaveName=ScopeData4
  adding_the_fuselage transmission_term_to the_const_term : Sum
  const_term fuselage_part : Product  Inputs=***//
  const_term pass_part : Product  Inputs=**//
  t_cab_term : Product  Inputs=**//
  t_cab_term_01 : Product  Inputs=**
  t_cab_term_02 : Product  Inputs=**
  t_cab_term_03 : Product  Inputs=**
  t_sa_term : Product  Inputs=***//
  Cabin Temp. [C] : Outport
  wires:
  Amb Temp [K]/1 -> Kinetic Heating/1(Amb. Temp. K)
  Mach #/1 -> Kinetic Heating/2(Mach#)
  Kinetic Heating/1(Recovery Temp [K]) -> K_to_C/1
  Cabin mdot & mass/1 -> Bus Selector/1
  Air Props./1 -> Bus Selector1/1
  Sup. Air Temp [C]/1 -> Scope2/1, t_sa_term/1  "temp_sa_C"
  Bus Selector/1 -> Scope2/2, t_sa_term/2  "<m_dot_sa>"
  Bus Selector1/1 -> Scope2/3, t_sa_term/3  "<Cp_sa>"
  Bus Selector/2 -> const_term fuselage_part/4, const_term pass_part/4, Scope2/4, t_sa_term/4, t_cab_term/3  "<m_cab>"
  Bus Selector1/2 -> const_term fuselage_part/5, const_term pass_part/3, Scope2/5, t_sa_term/5, t_cab_term/4  "<Cp_cab>"
  Cabin Param./1 -> Bus Selector2/1
  Bus Selector2/1 -> const_term pass_part/1  "<n_pass>"
  Bus Selector2/2 -> const_term pass_part/2  "<q_pass_W>"
  Bus Selector/3 -> t_cab_term_01/1  "<m_dot_ra>"
  Bus Selector1/3 -> t_cab_term_01/2  "<Cp_ra>"
  Bus Selector/4 -> t_cab_term_02/1  "<m_dot_ea>"
  Bus Selector1/4 -> t_cab_term_02/2  "<Cp_ea>"
  t_cab_term_01/1 -> Add/1
  t_cab_term_02/1 -> Add/2
  t_sa_term/1 -> Scope/1, Add1/1
  t_cab_term/1 -> Scope1/1, Add1/2
  Add/1 -> t_cab_term/1
  Add1/1 -> Integrator/1  "dTcab/dt"
  Integrator/1 -> t_cab_term/2, Cabin Temp. [C]/1
  Fuselage_parameters1/1(Fuselage Parameters) -> Bus Selector3/1
  Bus Selector3/1 -> t_cab_term_03/1, const_term fuselage_part/1  "<area_m2>"
  Bus Selector3/2 -> t_cab_term_03/2, const_term fuselage_part/2  "<U_Wpm2K>"
  t_cab_term_03/1 -> Add/3
  const_term pass_part/1 -> adding_the_fuselage transmission_term_to the_const_term/1
  adding_the_fuselage transmission_term_to the_const_term/1 -> Add1/3
  const_term fuselage_part/1 -> adding_the_fuselage transmission_term_to the_const_term/2
  K_to_C/1 -> const_term fuselage_part/3

== system ECS_FOS/ECS/Cabin Zone/Cabin_parameters ==
  note: Assuming that the thermal capacity of the cabin (C_p_cab)
      | is only due to the cabin air, not accounting for the furniture or
      | structure
  Bus Creator : BusCreator  Inputs=7
  Cp(P,T)3 : Lookup_n-D  BreakpointsForDimension1=AirProp.P  BreakpointsForDimension2=AirProp.T  BreakpointsForDimension3=[1]  Table=AirProp.Cp_pt  RndMeth=Simplest  InputSameDT=on
  Nominal cabin press_kPa : Constant  Value=80
  Nominal cabin temp_K : Constant  Value=298
  RAR : Constant  Value=RAR
  V_cab : Constant  Value=V_cab
  V_dot_sa_pass : Constant  Value=Vdot_sa_pass
  n_pack : Constant
  n_pass : Constant  Value=n_pass
  q_pass : Constant  Value=q_pass
  Cabin Parameters : Outport
  wires:
  n_pass/1 -> Bus Creator/1  "n_pass"
  V_cab/1 -> Bus Creator/2  "V_cab_m^3"
  q_pass/1 -> Bus Creator/3  "q_pass_W"
  n_pack/1 -> Bus Creator/4  "n_pack"
  Cp(P,T)3/1 -> Bus Creator/5  "C_p_cab_JKg^-1K^-1"
  Bus Creator/1 -> Cabin Parameters/1
  V_dot_sa_pass/1 -> Bus Creator/6  "V_dot_sa_pass"
  RAR/1 -> Bus Creator/7  "RAR"
  Nominal cabin press_kPa/1 -> Cp(P,T)3/1
  Nominal cabin temp_K/1 -> Cp(P,T)3/2

== system ECS_FOS/ECS/Cabin Zone/m_dot_sa_required1 ==
  Cabin Param. : Inport
  Sup. Air Prop. : Inport  Port=2
  Bus Selector : BusSelector  OutputSignals=n_pass,V_dot_sa_pass,n_pack
  Bus Selector1 : BusSelector  OutputSignals=Rho_sa
  Display : Display
  Display1 : Display
  Divide : Product  Inputs=***/
  mdot SA Req. : Outport
  wires:
  Cabin Param./1 -> Bus Selector/1
  Sup. Air Prop./1 -> Bus Selector1/1
  Bus Selector/1 -> Divide/1  "<n_pass>"
  Bus Selector/2 -> Divide/2  "<V_dot_sa_pass>"
  Bus Selector1/1 -> Divide/3, Display1/1  "<Rho_sa>"
  Bus Selector/3 -> Divide/4  "<n_pack>"
  Divide/1 -> mdot SA Req./1, Display/1

== system ECS_FOS/ECS/FOHX Left Wing/HX_Calcs ==
  Inputs : Inport
  Bus Creator1 : BusCreator
  Bus Creator2 : BusCreator  Inputs=2
  Fluid 1 Heat Transfer Calculation : Subsystem  TreatAsAtomicUnit=on
  Fluid 2 Heat Transfer Calculation : Subsystem  TreatAsAtomicUnit=on
  Input Processing : Subsystem
  Out : Outport
  wires:
  Fluid 1 Heat Transfer Calculation/3(q_h) -> [q1]
  Fluid 1 Heat Transfer Calculation/2(T_out_h) -> [T1_out]
  Fluid 1 Heat Transfer Calculation/1(h_out_h) -> [h1_out]
  Bus Creator1/1 -> Out/1  "Outputs"
  [Inputs] -> Fluid 1 Heat Transfer Calculation/1(Inputs)
  Inputs/1 -> Input Processing/1(Inputs)  "Inputs"
  Input Processing/1(Processed_Inputs) -> [Inputs]
  Fluid 2 Heat Transfer Calculation/3(q_h) -> [q2]
  Fluid 2 Heat Transfer Calculation/2(T_out) -> [T2_out]
  Fluid 2 Heat Transfer Calculation/1(h_out) -> [h2_out]
  [Inputs] -> Fluid 2 Heat Transfer Calculation/1(Inputs)
  [q1] -> Bus Creator2/1
  [q2] -> Bus Creator2/2
  Bus Creator2/1 -> [q]
  [T2_out] -> Bus Creator1/4  "T2_out"
  [h1_out] -> Bus Creator1/1  "h1_out"
  [T1_out] -> Bus Creator1/2  "T1_out"
  [h2_out] -> Bus Creator1/3  "h2_out"

== system ECS_FOS/ECS/FOHX Right Wing/HX_Calcs ==
  Inputs : Inport
  Bus Creator1 : BusCreator
  Bus Creator2 : BusCreator  Inputs=2
  Fluid 1 Heat Transfer Calculation : Subsystem  TreatAsAtomicUnit=on
  Fluid 2 Heat Transfer Calculation : Subsystem  TreatAsAtomicUnit=on
  Input Processing : Subsystem
  Out : Outport
  wires:
  [h2_out] -> Bus Creator1/3  "h2_out"
  [T1_out] -> Bus Creator1/2  "T1_out"
  [h1_out] -> Bus Creator1/1  "h1_out"
  [T2_out] -> Bus Creator1/4  "T2_out"
  Bus Creator2/1 -> [q]
  [q2] -> Bus Creator2/2
  [q1] -> Bus Creator2/1
  [Inputs] -> Fluid 2 Heat Transfer Calculation/1(Inputs)
  Fluid 2 Heat Transfer Calculation/1(h_out) -> [h2_out]
  Fluid 2 Heat Transfer Calculation/2(T_out) -> [T2_out]
  Fluid 2 Heat Transfer Calculation/3(q_h) -> [q2]
  Input Processing/1(Processed_Inputs) -> [Inputs]
  Inputs/1 -> Input Processing/1(Inputs)  "Inputs"
  [Inputs] -> Fluid 1 Heat Transfer Calculation/1(Inputs)
  Bus Creator1/1 -> Out/1  "Outputs"
  Fluid 1 Heat Transfer Calculation/1(h_out_h) -> [h1_out]
  Fluid 1 Heat Transfer Calculation/2(T_out_h) -> [T1_out]
  Fluid 1 Heat Transfer Calculation/3(q_h) -> [q1]

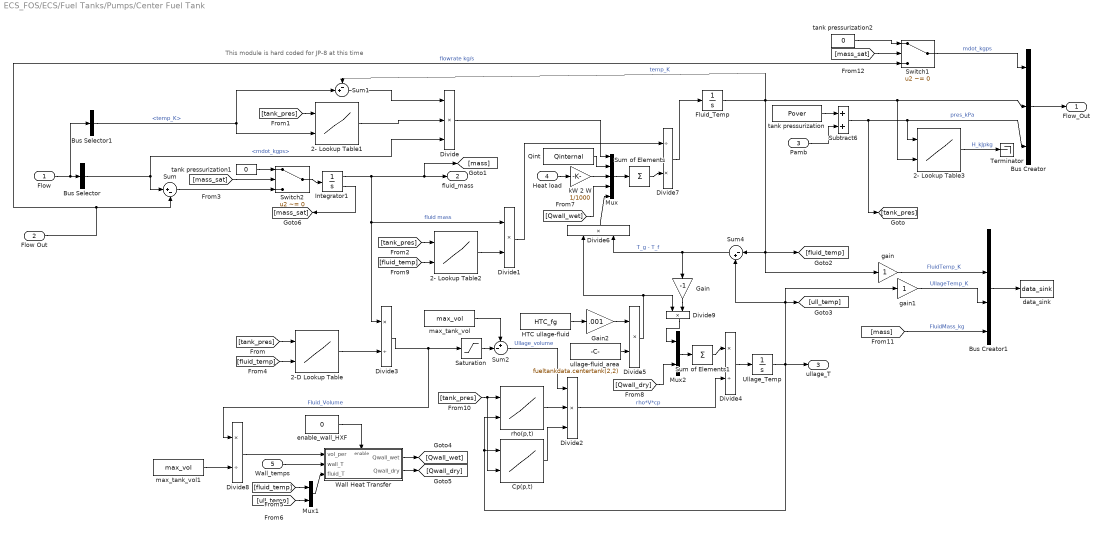
== system ECS_FOS/ECS/Fuel Tanks/Pumps/Center Fuel Tank ==
  note: This module is hard coded for JP-8 at this time
  Flow : Inport
  Flow Out : Inport  Port=2
  Pamb : Inport  Port=3
  Heat load : Inport  Port=4
  Wall_temps : Inport  Port=5
  2- Lookup Table1 : Lookup_n-D  BreakpointsForDimension1=F1.P  BreakpointsForDimension2=F1.T  Table=F1.Cp_pt  RndMeth=Simplest  InputSameDT=on
  2- Lookup Table2 : Lookup_n-D  BreakpointsForDimension1=F1.P  BreakpointsForDimension2=F1.T  Table=F1.Cp_pt  RndMeth=Simplest  InputSameDT=on
  2- Lookup Table3 : Lookup_n-D  BreakpointsForDimension1=F1.P  BreakpointsForDimension2=F1.T  Table=F1.H_pt  RndMeth=Simplest  InputSameDT=on
  2-D Lookup Table : Lookup_n-D  BreakpointsForDimension1=F1.P  BreakpointsForDimension2=F1.T  Table=F1.Rho_pt  RndMeth=Simplest  InputSameDT=on
  Bus Creator : BusCreator  Inputs=3
  Bus Creator1 : BusCreator
  Bus Selector : BusSelector  OutputSignals=mdot_kgps
  Bus Selector1 : BusSelector  OutputSignals=temp_K
  Cp(p,t) : Lookup_n-D  BreakpointsForDimension1=AirProp.P  BreakpointsForDimension2=AirProp.T  Table=AirProp.Cp_pt  RndMeth=Simplest  InputSameDT=on
  Divide : Product  Inputs=***
  Divide{1,5..6,9} (4 alike) : Product  Inputs=**
  Divide2 : Product  Inputs=***
  Divide3 : Product  Inputs=*/
  Divide4 : Product  Inputs=*/
  Divide7 : Product  Inputs=/*
  Divide8 : Product  Inputs=*/
  Fluid_Temp : Integrator  InitialCondition=fld_Tint + 273.15  LimitOutput=on  UpperSaturationLimit=800  LowerSaturationLimit=eps
  Gain : Gain  Gain=-1
  Gain2 : Gain  Gain=.001
  HTC ullage-fluid : Constant  Value=HTC_fg
  Integrator1 : Integrator  InitialCondition=m_init  LimitOutput=on  LowerSaturationLimit=1  ShowSaturationPort=on
  Mux : Mux  Inputs=5
  Mux1 : Mux  Inputs=2
  Mux2 : Mux  Inputs=2
  Qint : Constant  Value=Qinternal
  Saturation : Saturate  UpperLimit=inf  LowerLimit=eps  ZeroCross=off
  Subtract6 : Sum
  Sum : Sum  Inputs=|+-
  Sum of Elements : Sum  Inputs=+
  Sum of Elements1 : Sum  Inputs=+
  Sum1 : Sum  Inputs=-+|
  Sum2 : Sum  Inputs=+-|
  Sum4 : Sum  Inputs=|-+
  Switch1 : Switch  Criteria=u2 ~= 0  Threshold=-1
  Switch2 : Switch  Criteria=u2 ~= 0  Threshold=-1
  Terminator : Terminator
  Ullage_Temp : Integrator  InitialCondition=ull_Tint + 273.15  LimitOutput=on  LowerSaturationLimit=eps
  Wall Heat Transfer : Subsystem  TreatAsAtomicUnit=on
  data_sink : PowerFlowLib/Support Functions//Tools/data_sink
      link override global_data_goto: GotoTag=gdata_PowerFlowLibEnergyPowerSystemsThermalFuelFuelTank
  enable_wall_HXF : Constant  Value=0
  gain : Gain
  gain1 : Gain
  kW 2 W : Gain  Gain=1/1000
  max_tank_vol : Constant  Value=max_vol
  max_tank_vol1 : Constant  Value=max_vol
  rho(p,t) : Lookup_n-D  BreakpointsForDimension1=AirProp.P  BreakpointsForDimension2=AirProp.T  Table=AirProp.Rho_pt  RndMeth=Simplest  InputSameDT=on
  tank pressurization : Constant  Value=Pover
  tank pressurization1 : Constant  Value=0
  tank pressurization2 : Constant  Value=0
  ullage-fluid_area : Constant  Value=fueltankdata.centertank(2,2)
  Flow_Out : Outport
  fluid_mass : Outport  Port=2
  ullage_T : Outport  Port=3
  wires:
  Switch2/1 -> Integrator1/1
  tank pressurization1/1 -> Switch2/1
  [mass_sat] -> Switch2/2
  Integrator1/2 -> [mass_sat]
  Sum/1 -> Switch2/3
  tank pressurization2/1 -> Switch1/1
  [mass_sat] -> Switch1/2
  [mass] -> Bus Creator1/4  "FluidMass_kg"
  gain1/1 -> Bus Creator1/3  "UllageTemp_K"
  gain/1 -> Bus Creator1/2  "FluidTemp_K"
  Bus Creator1/1 -> data_sink/1
  kW 2 W/1 -> Mux/3
  2- Lookup Table3/1 -> Terminator/1  "H_kJpkg"
  Flow/1 -> Bus Selector/1, Bus Selector1/1
  Bus Selector/1 -> Divide/3, Sum/1  "<mdot_kgps>"
  Flow Out/1 -> Sum/2, Switch1/3  "flowrate kg/s"
  Integrator1/1 -> fluid_mass/1, [mass], Divide3/1, Divide1/1  "fluid mass"
  Bus Selector1/1 -> Sum1/2, 2- Lookup Table1/2  "<temp_K>"
  Sum1/1 -> Divide/1
  2- Lookup Table2/1 -> Divide1/2
  rho(p,t)/1 -> Divide2/2
  Cp(p,t)/1 -> Divide2/3
  Divide3/1 -> Saturation/1, Divide8/1  "Fluid_Volume"
  max_tank_vol/1 -> Sum2/1
  Sum2/1 -> Divide2/1  "Ullage_volume"
  Divide4/1 -> Ullage_Temp/1
  Ullage_Temp/1 -> ullage_T/1, gain1/1, Sum4/2, [ull_temp], rho(p,t)/2, Cp(p,t)/1
  Fluid_Temp/1 -> 2- Lookup Table3/2, Bus Creator/2, Sum1/1, gain/1, Sum4/1, [fluid_temp]  "temp_K"
  HTC ullage-fluid/1 -> Gain2/1
  ullage-fluid_area/1 -> Divide5/2
  Sum4/1 -> Divide6/2, Gain/1  "T_g - T_f"
  Divide1/1 -> Divide7/1
  Divide7/1 -> Fluid_Temp/1
  Divide5/1 -> Divide6/1, Divide9/1
  Pamb/1 -> Subtract6/2
  tank pressurization/1 -> Subtract6/1
  Subtract6/1 -> 2- Lookup Table3/1, Bus Creator/3, [tank_pres]  "pres_kPa"
  Bus Creator/1 -> Flow_Out/1
  Saturation/1 -> Sum2/2
  [tank_pres] -> 2-D Lookup Table/1
  2-D Lookup Table/1 -> Divide3/2
  [tank_pres] -> 2- Lookup Table1/1
  2- Lookup Table1/1 -> Divide/2
  [tank_pres] -> 2- Lookup Table2/1
  max_tank_vol1/1 -> Divide8/2
  Switch1/1 -> Bus Creator/1  "mdot_kgps"
  Divide/1 -> Mux/1
  Qint/1 -> Mux/2
  Heat load/1 -> kW 2 W/1
  Sum of Elements/1 -> Divide7/2
  Mux/1 -> Sum of Elements/1
  [fluid_temp] -> 2-D Lookup Table/2
  Divide8/1 -> Wall Heat Transfer/1(vol_per)
  Wall_temps/1 -> Wall Heat Transfer/2(wall_T)
  [fluid_temp] -> Mux1/1
  [ull_temp] -> Mux1/2
  Mux1/1 -> Wall Heat Transfer/3(fluid_T)
  Wall Heat Transfer/1(Qwall_wet) -> [Qwall_wet]
  Wall Heat Transfer/2(Qwall_dry) -> [Qwall_dry]
  Divide6/1 -> Mux/5
  Divide2/1 -> Divide4/2  "rho*V*cp"
  Mux2/1 -> Sum of Elements1/1
  Sum of Elements1/1 -> Divide4/1
  Gain/1 -> Divide9/2
  Divide9/1 -> Mux2/1
  [Qwall_dry] -> Mux2/2
  [Qwall_wet] -> Mux/4
  [fluid_temp] -> 2- Lookup Table2/2
  enable_wall_HXF/1 -> Wall Heat Transfer/Enable
  Gain2/1 -> Divide5/1
  [tank_pres] -> rho(p,t)/1, Cp(p,t)/2

== system ECS_FOS/ECS/Fuel Tanks/Pumps/FlowGenerator1 ==
  Bias : Bias  Bias=273.15
  Bus Creator1 : BusCreator
  Constant3 : Constant  Value=flowenthalpy
  Constant5 : Constant  Value=flowrate
  Constant6 : Constant  Value=flowtemp
  Constant7 : Constant  Value=flowpres
  FlowOut : Outport  Tag=Flow Out
  wires:
  Bus Creator1/1 -> FlowOut/1  "Outlet"
  Constant6/1 -> Bias/1  "temp_C"
  Constant7/1 -> Bus Creator1/3  "pres_kPa"
  Constant3/1 -> Bus Creator1/4  "H_kJpkg"
  Constant5/1 -> Bus Creator1/1  "mdot_kgps"
  Bias/1 -> Bus Creator1/2  "temp_K"

== system ECS_FOS/ECS/Fuel Tanks/Pumps/Fuel Control Left Wing ==
  FuelNeed : Inport
  FuelFromPump : Inport  Port=2
  Bus Creator : BusCreator  Inputs=3
  Bus Creator1 : BusCreator  Inputs=3
  Bus Selector : BusSelector  OutputSignals=mdot_kgps,temp_K,pres_kPa
  Gain : Gain
  Gain1 : Gain
  Saturation : Saturate  UpperLimit=inf  LowerLimit=0
  Sum : Sum  Inputs=|+-
  Switch : Switch  Criteria=u2 > Threshold
  Fuel2Engine : Outport
  Fuel2Tank : Outport  Port=2
  wires:
  FuelFromPump/1 -> Bus Selector/1
  Bus Selector/1 -> Sum/1, Switch/3  "<mdot_kgps>"
  FuelNeed/1 -> Sum/2, Switch/1
  Sum/1 -> Saturation/1, Switch/2
  Bus Creator/1 -> Fuel2Tank/1
  Bus Selector/2 -> Bus Creator/2, Gain1/1  "<temp_K>"
  Saturation/1 -> Bus Creator/1  "mdot_kgps"
  Switch/1 -> Bus Creator1/1  "mdot_kgps"
  Bus Selector/3 -> Bus Creator/3, Gain/1  "<pres_kPa>"
  Bus Creator1/1 -> Fuel2Engine/1
  Gain/1 -> Bus Creator1/3  "pres_kPa"
  Gain1/1 -> Bus Creator1/2  "temp_K"
